simulink model "actividad1"  (R2021a)
settings: Solver=ode1  StartTime=0.0  StopTime=10.0  FixedStep=0.0001  RelTol=1e-3
settings Model: Creator=valen  LastModifiedBy=valen

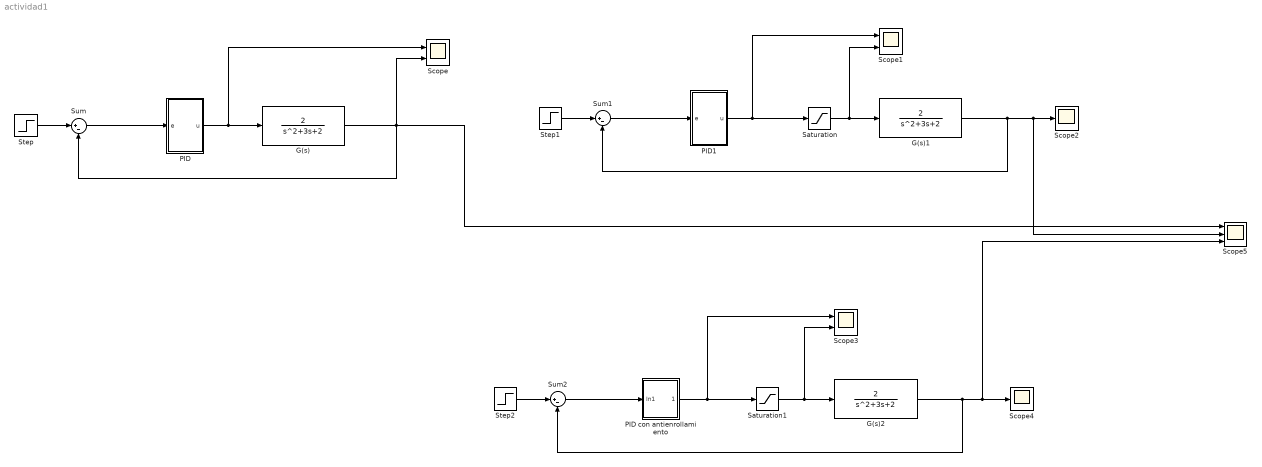
== system actividad1 ==
  G(s) : TransferFcn  Numerator=[2]  Denominator=[1 3 2]
  G(s)1 : TransferFcn  Numerator=[2]  Denominator=[1 3 2]
  G(s)2 : TransferFcn  Numerator=[2]  Denominator=[1 3 2]
  PID : Subsystem  mask{KP=5.67, KI=8, KD=0.93, tau=1/9.09}
  PID con antienrollamiento : Subsystem  mask{KP=5.67, KI=8, KD=0.93, tau=1/9.09, Umax=1, Umin=-1}
  PID1 : Subsystem  mask{KP=5.67, KI=8, KD=0.93, tau=1/9.09}
  Saturation : Saturate  UpperLimit=1  LowerLimit=-1
  Saturation1 : Saturate  UpperLimit=1  LowerLimit=-1
  Scope : Scope  NumInputPorts=2
  Scope1 : Scope  NumInputPorts=2
  Scope2 : Scope
  Scope3 : Scope  NumInputPorts=2
  Scope4 : Scope
  Scope5 : Scope  NumInputPorts=3
  Step : Step  After=0.8  SampleTime=0
  Step1 : Step  After=0.8  SampleTime=0
  Step2 : Step  After=0.8  SampleTime=0
  Sum : Sum  Inputs=|+-
  Sum1 : Sum  Inputs=|+-
  Sum2 : Sum  Inputs=|+-
  wires:
  Sum/1 -> PID/1(e)
  PID/1(u) -> Scope/1, G(s)/1
  Step/1 -> Sum/1
  G(s)/1 -> Scope/2, Scope5/1, Sum/2
  Sum1/1 -> PID1/1(e)
  Step1/1 -> Sum1/1
  PID1/1(u) -> Saturation/1, Scope1/1
  Saturation/1 -> G(s)1/1, Scope1/2
  G(s)1/1 -> Sum1/2, Scope5/2, Scope2/1
  Saturation1/1 -> G(s)2/1, Scope3/2
  G(s)2/1 -> Sum2/2, Scope5/3, Scope4/1
  Step2/1 -> Sum2/1
  Sum2/1 -> PID con antienrollamiento/1(In1)
  PID con antienrollamiento/1(Out1) -> Saturation1/1, Scope3/1

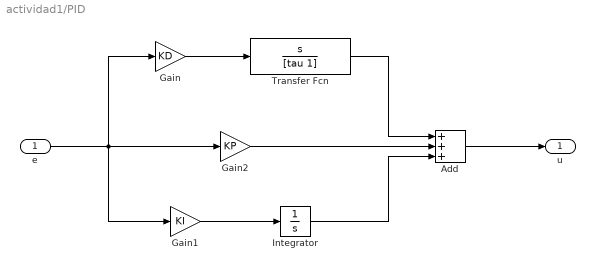
== system actividad1/PID ==
  e : Inport
  Add : Sum  Inputs=+++
  Gain : Gain  Gain=KD
  Gain1 : Gain  Gain=KI
  Gain2 : Gain  Gain=KP
  Integrator : Integrator
  Transfer Fcn : TransferFcn  Numerator=[1 0]  Denominator=[tau 1]
  u : Outport
  wires:
  Gain2/1 -> Add/2
  Integrator/1 -> Add/3
  e/1 -> Gain1/1, Gain2/1, Gain/1
  Transfer Fcn/1 -> Add/1
  Add/1 -> u/1
  Gain1/1 -> Integrator/1
  Gain/1 -> Transfer Fcn/1

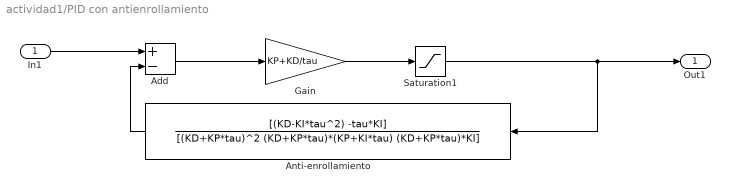
== system actividad1/PID con antienrollamiento ==
  In1 : Inport
  Add : Sum  Inputs=+-
  Anti-enrollamiento : TransferFcn  Numerator=[(KD-KI*tau^2) -tau*KI]  Denominator=[(KD+KP*tau)^2 (KD+KP*tau)*(KP+KI*tau) (KD+KP*tau)*KI]
  Gain : Gain  Gain=KP+KD/tau
  Saturation1 : Saturate  UpperLimit=Umax  LowerLimit=Umin
  Out1 : Outport
  wires:
  Anti-enrollamiento/1 -> Add/2
  Add/1 -> Gain/1
  Saturation1/1 -> Out1/1, Anti-enrollamiento/1
  In1/1 -> Add/1
  Gain/1 -> Saturation1/1

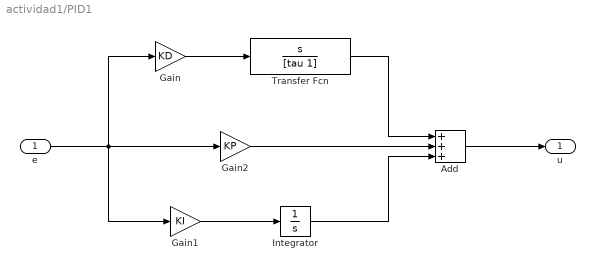
== system actividad1/PID1 ==
  e : Inport
  Add : Sum  Inputs=+++
  Gain : Gain  Gain=KD
  Gain1 : Gain  Gain=KI
  Gain2 : Gain  Gain=KP
  Integrator : Integrator
  Transfer Fcn : TransferFcn  Numerator=[1 0]  Denominator=[tau 1]
  u : Outport
  wires:
  Gain2/1 -> Add/2
  Integrator/1 -> Add/3
  e/1 -> Gain1/1, Gain2/1, Gain/1
  Transfer Fcn/1 -> Add/1
  Add/1 -> u/1
  Gain1/1 -> Integrator/1
  Gain/1 -> Transfer Fcn/1
